simulink model "Ejercicio19_20_02_17"  (R2013a)
settings: Solver=ode45  StartTime=0.0  StopTime=100  RelTol=1e-3
settings Model: Creator=Miguel  LastModifiedBy=Miguel

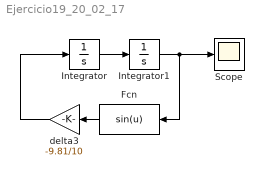
== system Ejercicio19_20_02_17 ==
  Fcn : Fcn  Expr=sin(u)
  Integrator : Integrator
  Integrator1 : Integrator  InitialCondition=pi/4
  Scope : Scope
      settings: ShowLegends=on  TimeRange=10
  delta3 : Gain  Gain=-9.81/10
  wires:
  Integrator1/1 -> Scope/1, Fcn/1
  Integrator/1 -> Integrator1/1
  Fcn/1 -> delta3/1
  delta3/1 -> Integrator/1
